simulink library "gm_combinedTxRx_ExternalMode_lib_org"  (Simulink 10.0)
settings: Solver=VariableStepAuto  StartTime=0.0  StopTime=10.0  RelTol=1e-3
undefined symbols (not defined in the file): AXI4, ip, Lite
libraries: axiinterfacelib x13
settings Model: Creator=tcollins  LastModifiedBy=bhisma

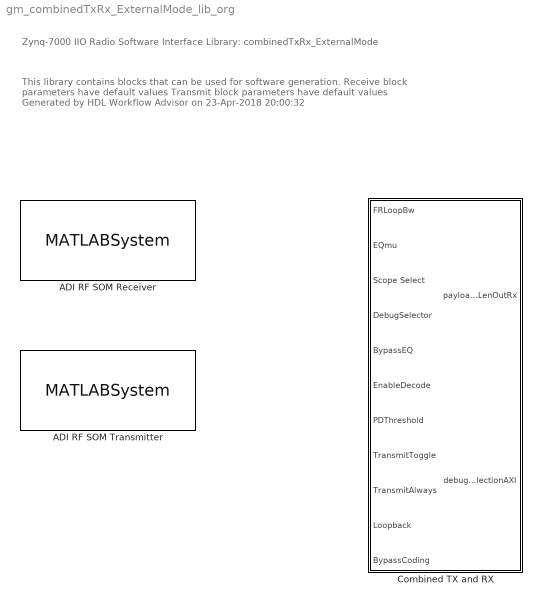
== system gm_combinedTxRx_ExternalMode_lib_org ==
  note: Zynq-7000 IIO Radio Software Interface Library: combinedTxRx_ExternalMode
  note: This library contains blocks that can be used for software generation.
      |
      | Receive block parameters have default values
      | Transmit block parameters have default values
      |
      | Generated by HDL Workflow Advisor on 23-Apr-2018 20:00:32
  ADI RF SOM Receiver : MATLABSystem  System=comm.SDRRxZynqRadioLibIIO  IPAddress=192.168.3.2  uri=ip:10.0.0.200  CenterFrequencySource=Dialog  CenterFrequency=2.4e9  GainSource=AGC Slow Attack  Gain=10  ChannelMapping=1  BasebandSampleRate=1e6  OutputDataType=int16  SamplesPerFrame=20000  OverflowOutputPort=on  ShowAdvancedProperties=off  Timeout=30  EnableQuadratureTracking=on  EnableRFDCTracking=on  EnableBasebandDCTracking=on  UseCustomFilter=off  filtPathRates=[ 737280000, 11520000, 3840000, 1920000, 960000, 240000 ]  filtCoefficients=round( fir1( 127, 0.75 )*2^15*10^1.2 )  filtCoefficientSize=128  filtDecimInterpFactor=4  filtGain=-12  filtRFBandwidth=18e6  filterConfigStruct=struct()  ENSMPinControlMode=None  BISTLoopbackMode=Disabled
      mask Type: comm.SDRRxZynqRadioLibIIO
      mask Display:
      | disp(['SDR' char(10) 'Receiver']);
      | port_label('output',1,'data');
      | port_label('output',2,'data valid');
      | port_label('output',3,'overflow');
  ADI RF SOM Transmitter : MATLABSystem  System=comm.SDRTxZynqRadioLibIIO  IPAddress=192.168.3.2  uri=ip:10.0.0.200  CenterFrequencySource=Dialog  CenterFrequency=2.4e9  GainSource=Dialog  Gain=-10  ChannelMapping=1  BasebandSampleRate=1e6  UnderflowOutputPort=on  ShowAdvancedProperties=off  Timeout=30  DataSourceSelect=Input Port  DDSTone1Freq=5e3  DDSTone2Freq=10e3  DDSTone1Scale=0.5  DDSTone2Scale=0.25  UseCustomFilter=off  filtPathRates=[ 737280000, 11520000, 3840000, 1920000, 960000, 240000 ]  filtCoefficients=round( fir1( 127, 0.75 )*2^15*10^1.2 )  filtCoefficientSize=128  filtDecimInterpFactor=4  filtGain=-12  filtRFBandwidth=18e6  filterConfigStruct=struct()  ENSMPinControlMode=None  BISTLoopbackMode=Disabled
      mask Type: comm.SDRTxZynqRadioLibIIO
      mask Display:
      | disp(['SDR' char(10) 'Transmitter']);
      | port_label('input',1,'data');
      | port_label('output',1,'underflow');
  Combined TX and RX : Subsystem  TreatAsAtomicUnit=on  mask(AXI4-Lite/AXI4 Interface){}
      mask help:
      | This is an automatically generated subsystem block.
      | This contains the AXI interface blocks that communicate with the CombinedT_ip IPCore generated from combinedTxRx_ExternalMode/Combined TX and RX subsystem.
      mask Display: disp(sprintf('Xilinx Zynq \nAXI Interface'));

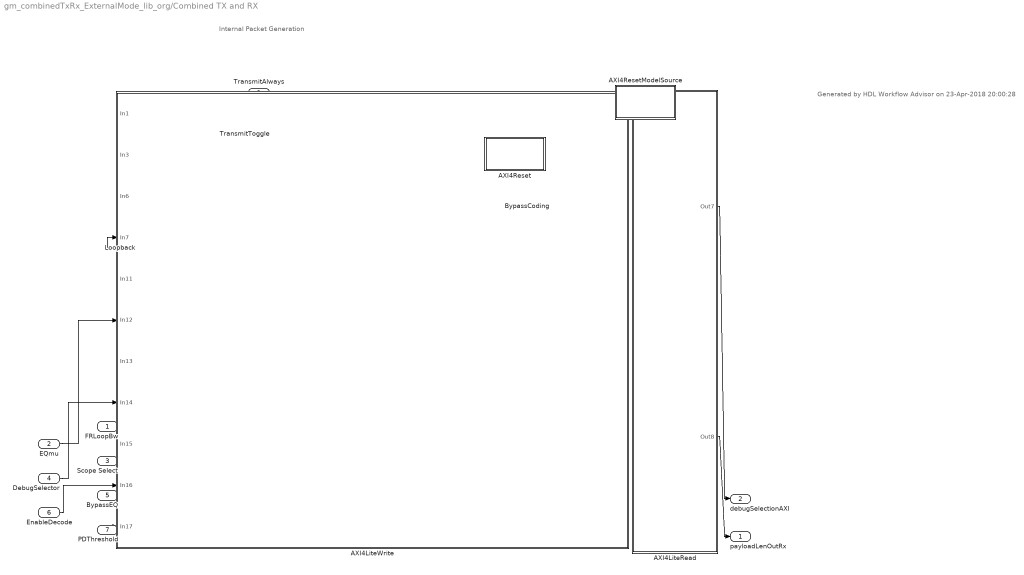
== system gm_combinedTxRx_ExternalMode_lib_org/Combined TX and RX ==
  note: Generated by HDL Workflow Advisor on 23-Apr-2018 20:00:28
  note: Internal Packet Generation
  FRLoopBw : Inport
  EQmu : Inport  Port=2
  Scope Select : Inport  Port=3
  DebugSelector : Inport  Port=4
  BypassEQ : Inport  Port=5
  EnableDecode : Inport  Port=6
  PDThreshold : Inport  Port=7
  TransmitToggle : Inport  Port=8
  TransmitAlways : Inport  Port=9
  Loopback : Inport  Port=10
  BypassCoding : Inport  Port=11
  AXI4LiteRead : Subsystem  Priority=10
  AXI4LiteWrite : Subsystem  Priority=1
  AXI4Reset : Subsystem  mask(System Start){ShowInLibBrowser=0}
      mask prompts: ShowInLibBrowser "Simulink:masks:CustCodeMaskParam1_MP"
      settings: CopyFcn=cccopyfcn(gcb)  OpenFcn=ccopenfcn('System Start Function')
      mask Help: eval('feval(''rtwprivate'',''rtwhelpview'',''rtw_sys_start_block'')');
      mask Display: disp('System\nStart');
  AXI4ResetModelSource : Subsystem  mask(Model Source){ShowInLibBrowser=0}
      mask prompts: ShowInLibBrowser "Simulink:masks:CustCodeMaskParam1_MP"
      settings: CopyFcn=cccopyfcn(gcb)  OpenFcn=ccopenfcn('Model Source')
      mask Help: eval('feval(''rtwprivate'',''rtwhelpview'',''rtw_model_source_block'')');
      mask Display: disp('Model\nSource');
  payloadLenOutRx : Outport  VectorParamsAs1DForOutWhenUnconnected=off
  debugSelectionAXI : Outport  Port=2  VectorParamsAs1DForOutWhenUnconnected=off
  wires:
  AXI4LiteRead/2(Out8) -> payloadLenOutRx/1
  AXI4LiteRead/1(Out7) -> debugSelectionAXI/1
  PDThreshold/1 -> AXI4LiteWrite/11(In17)
  EnableDecode/1 -> AXI4LiteWrite/10(In16)
  BypassEQ/1 -> AXI4LiteWrite/9(In15)
  DebugSelector/1 -> AXI4LiteWrite/8(In14)
  Scope Select/1 -> AXI4LiteWrite/7(In13)
  EQmu/1 -> AXI4LiteWrite/6(In12)
  FRLoopBw/1 -> AXI4LiteWrite/5(In11)
  Loopback/1 -> AXI4LiteWrite/4(In7)
  BypassCoding/1 -> AXI4LiteWrite/3(In6)
  TransmitToggle/1 -> AXI4LiteWrite/2(In3)
  TransmitAlways/1 -> AXI4LiteWrite/1(In1)

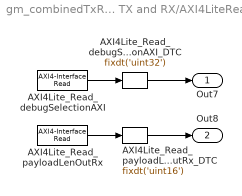
== system gm_combinedTxRx_ExternalMode_lib_org/Combined TX and RX/AXI4LiteRead ==
  AXI4Lite_Read_debugSelectionAXI : axiinterfacelib/AXI4-Interface Read  Priority=9  AXIInterfaceType=AXI4-Lite  DeviceName=/dev/mwipcore  RegisterOffset=hex2dec('140')  DataLength=1  DataType=uint32  SampleTime=-1  blockPlatform=ZYNQ  SimulateUsing=Interpreted Execution
      settings: SourceProductName=Embedded Coder Support Package for Xilinx Zynq Platform  SourceProductBaseCode=ECZYNQ7000
  AXI4Lite_Read_debugSelectionAXI_DTC : DataTypeConversion  OutDataTypeStr=fixdt('uint32')  ConvertRealWorld=Stored Integer (SI)
  AXI4Lite_Read_payloadLenOutRx : axiinterfacelib/AXI4-Interface Read  Priority=8  AXIInterfaceType=AXI4-Lite  DeviceName=/dev/mwipcore  RegisterOffset=hex2dec('110')  DataLength=1  DataType=uint32  SampleTime=-1  blockPlatform=ZYNQ  SimulateUsing=Interpreted Execution
      settings: SourceProductName=Embedded Coder Support Package for Xilinx Zynq Platform  SourceProductBaseCode=ECZYNQ7000
  AXI4Lite_Read_payloadLenOutRx_DTC : DataTypeConversion  OutDataTypeStr=fixdt('uint16')  ConvertRealWorld=Stored Integer (SI)
  Out7 : Outport  VectorParamsAs1DForOutWhenUnconnected=off
  Out8 : Outport  Port=2  VectorParamsAs1DForOutWhenUnconnected=off
  wires:
  AXI4Lite_Read_debugSelectionAXI/1 -> AXI4Lite_Read_debugSelectionAXI_DTC/1
  AXI4Lite_Read_debugSelectionAXI_DTC/1 -> Out7/1
  AXI4Lite_Read_payloadLenOutRx/1 -> AXI4Lite_Read_payloadLenOutRx_DTC/1
  AXI4Lite_Read_payloadLenOutRx_DTC/1 -> Out8/1

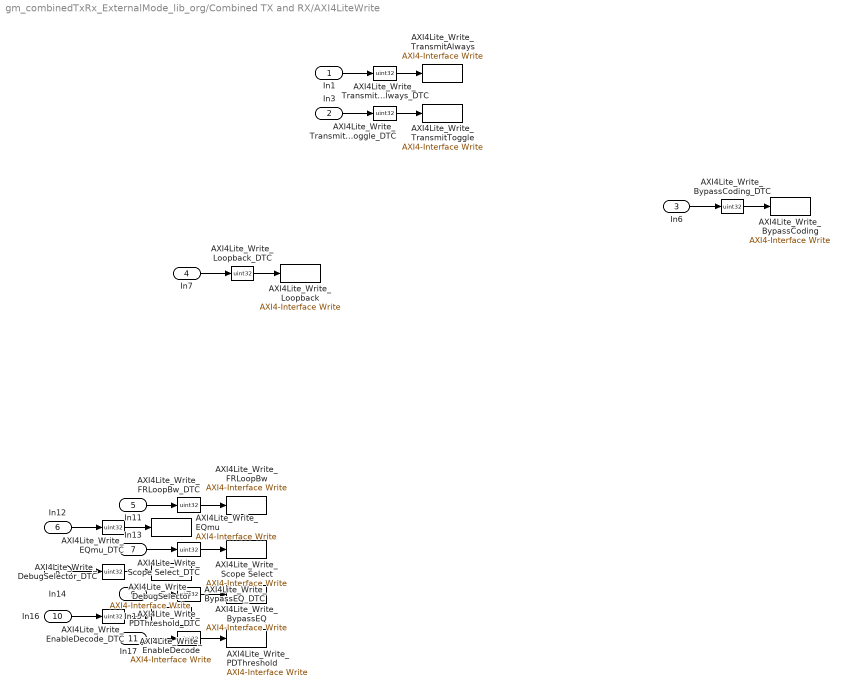
== system gm_combinedTxRx_ExternalMode_lib_org/Combined TX and RX/AXI4LiteWrite ==
  In1 : Inport
  In3 : Inport  Port=2
  In6 : Inport  Port=3
  In7 : Inport  Port=4
  In11 : Inport  Port=5
  In12 : Inport  Port=6
  In13 : Inport  Port=7
  In14 : Inport  Port=8
  In15 : Inport  Port=9
  In16 : Inport  Port=10
  In17 : Inport  Port=11
  AXI4Lite_Write_BypassCoding : axiinterfacelib/AXI4-Interface Write  Priority=17  AXIInterfaceType=AXI4-Lite  DeviceName=/dev/mwipcore  RegisterOffset=hex2dec('130')  blockPlatform=ZYNQ  SimulateUsing=Interpreted execution
      settings: SourceProductName=Embedded Coder Support Package for Xilinx Zynq Platform  SourceProductBaseCode=ECZYNQ7000
  AXI4Lite_Write_BypassCoding_DTC : DataTypeConversion  OutDataTypeStr=uint32  ConvertRealWorld=Stored Integer (SI)
  AXI4Lite_Write_BypassEQ : axiinterfacelib/AXI4-Interface Write  Priority=11  AXIInterfaceType=AXI4-Lite  DeviceName=/dev/mwipcore  RegisterOffset=hex2dec('114')  blockPlatform=ZYNQ  SimulateUsing=Interpreted execution
      settings: SourceProductName=Embedded Coder Support Package for Xilinx Zynq Platform  SourceProductBaseCode=ECZYNQ7000
  AXI4Lite_Write_BypassEQ_DTC : DataTypeConversion  OutDataTypeStr=uint32  ConvertRealWorld=Stored Integer (SI)
  AXI4Lite_Write_DebugSelector : axiinterfacelib/AXI4-Interface Write  Priority=10  AXIInterfaceType=AXI4-Lite  DeviceName=/dev/mwipcore  RegisterOffset=hex2dec('10C')  blockPlatform=ZYNQ  SimulateUsing=Interpreted execution
      settings: SourceProductName=Embedded Coder Support Package for Xilinx Zynq Platform  SourceProductBaseCode=ECZYNQ7000
  AXI4Lite_Write_DebugSelector_DTC : DataTypeConversion  OutDataTypeStr=uint32  ConvertRealWorld=Stored Integer (SI)
  AXI4Lite_Write_EQmu : axiinterfacelib/AXI4-Interface Write  Priority=8  AXIInterfaceType=AXI4-Lite  DeviceName=/dev/mwipcore  RegisterOffset=hex2dec('104')  blockPlatform=ZYNQ  SimulateUsing=Interpreted execution
      settings: SourceProductName=Embedded Coder Support Package for Xilinx Zynq Platform  SourceProductBaseCode=ECZYNQ7000
  AXI4Lite_Write_EQmu_DTC : DataTypeConversion  OutDataTypeStr=uint32  ConvertRealWorld=Stored Integer (SI)
  AXI4Lite_Write_EnableDecode : axiinterfacelib/AXI4-Interface Write  Priority=12  AXIInterfaceType=AXI4-Lite  DeviceName=/dev/mwipcore  RegisterOffset=hex2dec('118')  blockPlatform=ZYNQ  SimulateUsing=Interpreted execution
      settings: SourceProductName=Embedded Coder Support Package for Xilinx Zynq Platform  SourceProductBaseCode=ECZYNQ7000
  AXI4Lite_Write_EnableDecode_DTC : DataTypeConversion  OutDataTypeStr=uint32  ConvertRealWorld=Stored Integer (SI)
  AXI4Lite_Write_FRLoopBw : axiinterfacelib/AXI4-Interface Write  Priority=7  AXIInterfaceType=AXI4-Lite  DeviceName=/dev/mwipcore  RegisterOffset=hex2dec('100')  blockPlatform=ZYNQ  SimulateUsing=Interpreted execution
      settings: SourceProductName=Embedded Coder Support Package for Xilinx Zynq Platform  SourceProductBaseCode=ECZYNQ7000
  AXI4Lite_Write_FRLoopBw_DTC : DataTypeConversion  OutDataTypeStr=uint32  ConvertRealWorld=Stored Integer (SI)
  AXI4Lite_Write_Loopback : axiinterfacelib/AXI4-Interface Write  Priority=16  AXIInterfaceType=AXI4-Lite  DeviceName=/dev/mwipcore  RegisterOffset=hex2dec('12C')  blockPlatform=ZYNQ  SimulateUsing=Interpreted execution
      settings: SourceProductName=Embedded Coder Support Package for Xilinx Zynq Platform  SourceProductBaseCode=ECZYNQ7000
  AXI4Lite_Write_Loopback_DTC : DataTypeConversion  OutDataTypeStr=uint32  ConvertRealWorld=Stored Integer (SI)
  AXI4Lite_Write_PDThreshold : axiinterfacelib/AXI4-Interface Write  Priority=13  AXIInterfaceType=AXI4-Lite  DeviceName=/dev/mwipcore  RegisterOffset=hex2dec('11C')  blockPlatform=ZYNQ  SimulateUsing=Interpreted execution
      settings: SourceProductName=Embedded Coder Support Package for Xilinx Zynq Platform  SourceProductBaseCode=ECZYNQ7000
  AXI4Lite_Write_PDThreshold_DTC : DataTypeConversion  OutDataTypeStr=uint32  ConvertRealWorld=Stored Integer (SI)
  AXI4Lite_Write_Scope Select : axiinterfacelib/AXI4-Interface Write  Priority=9  AXIInterfaceType=AXI4-Lite  DeviceName=/dev/mwipcore  RegisterOffset=hex2dec('108')  blockPlatform=ZYNQ  SimulateUsing=Interpreted execution
      settings: SourceProductName=Embedded Coder Support Package for Xilinx Zynq Platform  SourceProductBaseCode=ECZYNQ7000
  AXI4Lite_Write_Scope Select_DTC : DataTypeConversion  OutDataTypeStr=uint32  ConvertRealWorld=Stored Integer (SI)
  AXI4Lite_Write_TransmitAlways : axiinterfacelib/AXI4-Interface Write  Priority=15  AXIInterfaceType=AXI4-Lite  DeviceName=/dev/mwipcore  RegisterOffset=hex2dec('124')  blockPlatform=ZYNQ  SimulateUsing=Interpreted execution
      settings: SourceProductName=Embedded Coder Support Package for Xilinx Zynq Platform  SourceProductBaseCode=ECZYNQ7000
  AXI4Lite_Write_TransmitAlways_DTC : DataTypeConversion  OutDataTypeStr=uint32  ConvertRealWorld=Stored Integer (SI)
  AXI4Lite_Write_TransmitToggle : axiinterfacelib/AXI4-Interface Write  Priority=14  AXIInterfaceType=AXI4-Lite  DeviceName=/dev/mwipcore  RegisterOffset=hex2dec('120')  blockPlatform=ZYNQ  SimulateUsing=Interpreted execution
      settings: SourceProductName=Embedded Coder Support Package for Xilinx Zynq Platform  SourceProductBaseCode=ECZYNQ7000
  AXI4Lite_Write_TransmitToggle_DTC : DataTypeConversion  OutDataTypeStr=uint32  ConvertRealWorld=Stored Integer (SI)
  wires:
  AXI4Lite_Write_FRLoopBw_DTC/1 -> AXI4Lite_Write_FRLoopBw/1
  In11/1 -> AXI4Lite_Write_FRLoopBw_DTC/1
  AXI4Lite_Write_BypassCoding_DTC/1 -> AXI4Lite_Write_BypassCoding/1
  In6/1 -> AXI4Lite_Write_BypassCoding_DTC/1
  AXI4Lite_Write_Loopback_DTC/1 -> AXI4Lite_Write_Loopback/1
  AXI4Lite_Write_TransmitAlways_DTC/1 -> AXI4Lite_Write_TransmitAlways/1
  In1/1 -> AXI4Lite_Write_TransmitAlways_DTC/1
  In7/1 -> AXI4Lite_Write_Loopback_DTC/1
  AXI4Lite_Write_TransmitToggle_DTC/1 -> AXI4Lite_Write_TransmitToggle/1
  In3/1 -> AXI4Lite_Write_TransmitToggle_DTC/1
  AXI4Lite_Write_PDThreshold_DTC/1 -> AXI4Lite_Write_PDThreshold/1
  In16/1 -> AXI4Lite_Write_EnableDecode_DTC/1
  In17/1 -> AXI4Lite_Write_PDThreshold_DTC/1
  AXI4Lite_Write_EnableDecode_DTC/1 -> AXI4Lite_Write_EnableDecode/1
  AXI4Lite_Write_BypassEQ_DTC/1 -> AXI4Lite_Write_BypassEQ/1
  In15/1 -> AXI4Lite_Write_BypassEQ_DTC/1
  In14/1 -> AXI4Lite_Write_DebugSelector_DTC/1
  AXI4Lite_Write_DebugSelector_DTC/1 -> AXI4Lite_Write_DebugSelector/1
  AXI4Lite_Write_Scope Select_DTC/1 -> AXI4Lite_Write_Scope Select/1
  In13/1 -> AXI4Lite_Write_Scope Select_DTC/1
  In12/1 -> AXI4Lite_Write_EQmu_DTC/1
  AXI4Lite_Write_EQmu_DTC/1 -> AXI4Lite_Write_EQmu/1

== system gm_combinedTxRx_ExternalMode_lib_org/Combined TX and RX/AXI4Reset ==

== system gm_combinedTxRx_ExternalMode_lib_org/Combined TX and RX/AXI4ResetModelSource ==
